simulink model "EXP_GEN"  (R2018b)
settings: Solver=VariableStepAuto  StartTime=1  StopTime=10000  RelTol=1e-3
settings Model: Creator=maiabdelhakim  LastModifiedBy=yx46_

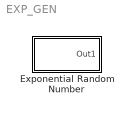
== system EXP_GEN ==
  Exponential Random Number : Subsystem  mask(Exponential Random Number){mean=1, seed=123}
      mask prompts: seed "Random Seed"
      mask help: This block generate a random number with exponential distribution.
      mask Display: disp(['mean=' num2str(mean,2)],"texmode","on");

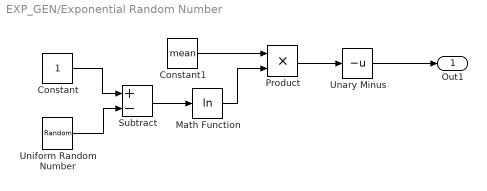
== system EXP_GEN/Exponential Random Number ==
  Constant : Constant
  Constant1 : Constant  Value=mean
  Math Function : Math  Operator=log  SaturateOnIntegerOverflow=on
  Product : Product  RndMeth=Zero
  Subtract : Sum  Inputs=+-
  Unary Minus : UnaryMinus
  Uniform Random Number : UniformRandomNumber  Minimum=0  Seed=seed
  Out1 : Outport
  wires:
  Subtract/1 -> Math Function/1
  Math Function/1 -> Product/2
  Unary Minus/1 -> Out1/1
  Product/1 -> Unary Minus/1
  Constant/1 -> Subtract/1
  Uniform Random Number/1 -> Subtract/2
  Constant1/1 -> Product/1
